simulink subsystem "newton"  (R2024b)
settings: Solver=VariableStepAuto  StartTime=0.0  StopTime=10.0  RelTol=1e-3
undefined symbols (not defined in the file): DiscIntNeverNeededParam, speed_init
settings Model: Creator=yagiz  LastModifiedBy=yagiz

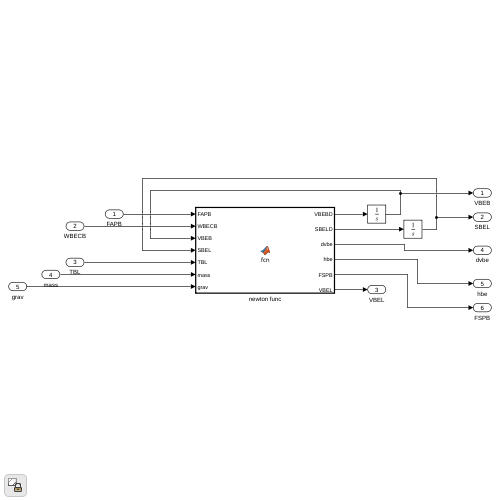
[thumbnail: Simulink's stored preview of the top-level diagram]
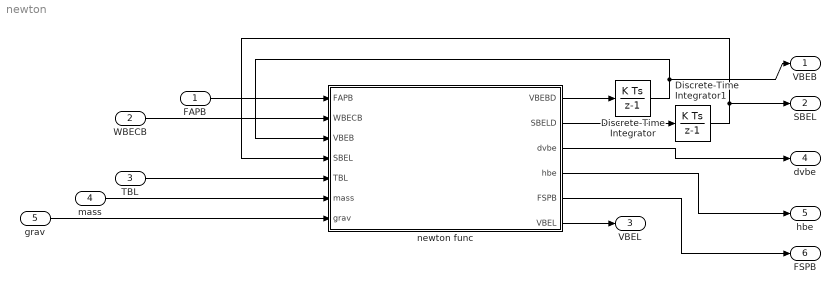
== system newton ==
  FAPB : Inport
  WBECB : Inport  Port=2
  TBL : Inport  Port=3
  mass : Inport  Port=4
  grav : Inport  Port=5
  Discrete-Time Integrator : DiscreteIntegrator  InitialCondition=[speed_init; 0; 0]  SampleTime=0.001  ICPrevOutput=DiscIntNeverNeededParam  ICPrevScaledInput=DiscIntNeverNeededParam
  Discrete-Time Integrator1 : DiscreteIntegrator  InitialCondition=sbel_init'  SampleTime=0.001  ICPrevOutput=DiscIntNeverNeededParam  ICPrevScaledInput=DiscIntNeverNeededParam
  newton func : MATLAB Function  TreatAsAtomicUnit=on
  VBEB : Outport
  SBEL : Outport  Port=2
  VBEL : Outport  Port=3
  dvbe : Outport  Port=4
  hbe : Outport  Port=5
  FSPB : Outport  Port=6
  wires:
  newton func/1(VBEBD) -> Discrete-Time Integrator/1
  Discrete-Time Integrator/1 -> VBEB/1, newton func/3(VBEB)
  newton func/2(SBELD) -> Discrete-Time Integrator1/1
  Discrete-Time Integrator1/1 -> newton func/4(SBEL), SBEL/1
  FAPB/1 -> newton func/1(FAPB)
  WBECB/1 -> newton func/2(WBECB)
  TBL/1 -> newton func/5(TBL)
  mass/1 -> newton func/6(mass)
  grav/1 -> newton func/7(grav)
  newton func/6(VBEL) -> VBEL/1
  newton func/5(FSPB) -> FSPB/1
  newton func/3(dvbe) -> dvbe/1
  newton func/4(hbe) -> hbe/1

== matlab function newton/newton func ==
  data: FAPB input; VBEBD output; WBECB input size=[3 1]; VBEB input; SBEL input; TBL input; mass input; grav input; SBELD output; dvbe output; hbe output; FSPB output; VBEL output
function [VBEBD, SBELD, dvbe, hbe, FSPB, VBEL] = fcn(FAPB, WBECB, VBEB, SBEL, TBL, mass, grav)

WBECB = WBECB(:);
VBEB  = VBEB(:);
FAPB  = FAPB(:);
SBEL  = SBEL(:);


% Specific force (body axes)
FSPB = FAPB / mass;

% Coriolis term
ATB = cross(WBECB, VBEB);

% Gravity in body axes (NED: gravity = +Down)
GRAVL = [0; 0; grav];
GRAVB = TBL * GRAVL;

% Body-frame velocity derivative
VBEBD = FSPB - ATB + GRAVB;

% NED velocity (transpose of TBL)
VBEL = TBL' * VBEB;

% Position derivative
SBELD = VBEL;

% Scalar speed and altitude
dvbe = norm(VBEL);
hbe  = -SBEL(3);
